simulink model "warning_system_harness"  (R2024b)
settings: Solver=FixedStepAuto  StartTime=0.0  StopTime=1500  FixedStep=TS_MODEL  RelTol=1e-3
InitFcn:
  | %run('config.m');
undefined symbols (not defined in the file or in its folder): THRESHOLD_CAUTION, THRESHOLD_CRASHED, THRESHOLD_LANE_CHANGE, THRESHOLD_REST, TS_CORE
libraries: dspstat3 x3, simulink x3, SignalEditorBlockLib x1
settings Model: DataDictionary=try__.sldd  SimulationMode=rapid-accelerator  ExtModeTrigDuration=2  Creator=Nitesh  LastModifiedBy=Nitesh
settings SolverCC: AutoInsertRateTranBlk=on
settings OptimizationCC: EnhancedBackFolding=on  PassReuseOutputArgsAs=Individual arguments  ZeroExternalMemoryAtStartup=off  ZeroInternalMemoryAtStartup=off  MaxStackSize=64  OptimizeBlockOrder=speed  DifferentSizesBufferReuse=on  OptimizationCustomize=off  EfficientTunableParamExpr=on
settings DebuggingCC: ParameterTunabilityLossMsg=error
settings HardwareCC: ProdBitPerPointer=32  ProdBitPerSizeT=32  ProdBitPerPtrDiffT=32  ProdLargestAtomicInteger=Long  ProdLargestAtomicFloat=Double  ProdWordSize=32  ProdHWDeviceType=ARM Compatible->ARM Cortex  UseEmbeddedCoderFeatures=off
settings RTWCC: Description=Embedded Coder  SystemTargetFile=ert.tlc  HardwareBoard=ESP32-WROOM(Arduino Compatible)  TLCOptions="-aInlineSetEventsForThisBaseRateFcn=TLC_FALSE -aSuppressMultiTaskScheduler=TLC_FALSE  -aRateBasedStepFcn=0"  TemplateMakefile=ert_default_tmf  Toolchain=ESP32
settings CodeAppCC: ForceParamTrailComments=on  IgnoreCustomStorageClasses=off  OperatorAnnotations=on  SimulinkDataObjDesc=on  SFDataObjDesc=on  InsertBlockDesc=on
settings ERTTargetCC: MultiwordLength=2048  DynamicStringBufferSize=2048  SupportContinuousTime=on  SupportNonInlinedSFcns=on  SupportVariableSizeSignals=on  ExtModeTransport=3  ExtModeStaticAlloc=on  ExtModeAutomaticAllocSize=off  ExtModeStaticAllocSize=65536  ExtModeMexFile=ext_xcp  ExtModeIntrfLevel=Level2 - Open  InlinedParameterPlacement=Hierarchical

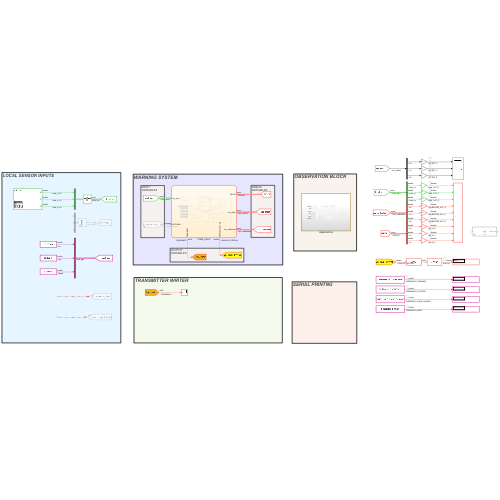
[thumbnail: Simulink's stored preview of the top-level diagram]
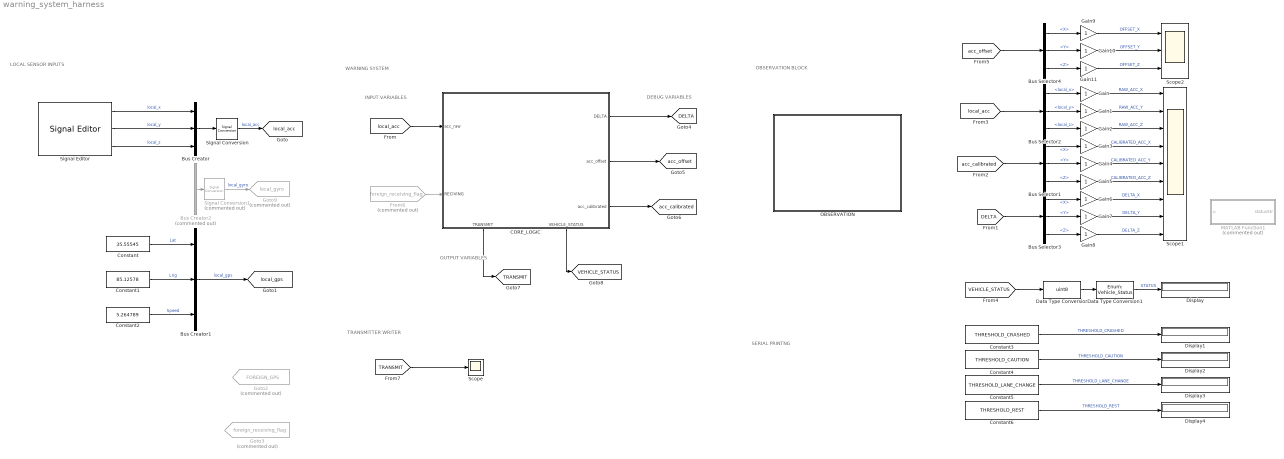
== system warning_system_harness ==
  note: SERIAL PRINTNG
  note: DEBUG
      | VARIABLES
  note: OBSERVATION BLOCK
  note: TRANSMITTER WRITER
  note: WARNING SYSTEM
  note: LOCAL SENSOR INPUTS
  note: OUTPUT
      | VARIABLES
  note: INPUT
      | VARIABLES
  Bus Creator : BusCreator  Inputs=3
  Bus Creator1 : BusCreator  Inputs=3
  Bus Creator2 : BusCreator  Commented=on  Inputs=3
  Bus Selector1 : BusSelector  OutputSignals=X,Y,Z
  Bus Selector2 : BusSelector  OutputSignals=local_x,local_y,local_z
  Bus Selector3 : BusSelector  OutputSignals=X,Y,Z
  Bus Selector4 : BusSelector  OutputSignals=X,Y,Z
  CORE_LOGIC : Stateflow chart  TreatAsAtomicUnit=on  SystemSampleTime=TS_CORE
      settings: PortSchema="{\"entries\":[{\"content\":{\"sides\":[{\"content\":{\"connectorIds\":[\"In2\",\"In1\"]},\"type\":\"ConnectorPlacement.EquallySpacedRectSide\",\"uuid\":\"ee7c9145-97fe-42bf-b38f-25095debb339\"},{\"content\":{\"connectorIds\":[\"Out2\",\"Out3\",\"Out4\"],\"side\":\"RIGHT\"},\"type\":\"ConnectorPlacement.EquallySpacedRectSide\",\"uuid\":\"6ad3cc48-74a8-47e1-8b84-b3331846d199\"},{\"content\":{\"side\":\"TOP\"},\"type\":\"ConnectorPlacement.EquallySpacedRectSide\",\"uuid\":\"0e80e778-40c2-414e-b172-27c343627a22\"},{\"content\":{\"connectorIds\":[\"Out1\",\"Out5\"],\"side\":\"BOTTOM\"},\"type\":\"ConnectorPlacement.EquallySpacedRectSide\",\"uuid\":\"8c076511-fb77-4abd-9a6c-f32e2686fd08\"}]},\"type\":\"ConnectorPlacement.EquallySpacedConnector\",\"uuid\":\"44f6d062-1c8f-4774-b93e-5476bfb914ed\"}],\"packageUris\":[\"http://schema.mathworks.com/mf0/Connector/R2020b\"],\"version\":\"1.0\"}"
  Constant : Constant  Value=35.55545
  Constant1 : Constant  Value=85.12578
  Constant2 : Constant  Value=5.264789
  Constant3 : Constant  Value=THRESHOLD_CRASHED
  Constant4 : Constant  Value=THRESHOLD_CAUTION
  Constant5 : Constant  Value=THRESHOLD_LANE_CHANGE
  Constant6 : Constant  Value=THRESHOLD_REST
  Data Type Conversion : DataTypeConversion  OutDataTypeStr=uint8  SaturateOnIntegerOverflow=off  RndMeth=Floor
  Data Type Conversion1 : DataTypeConversion  OutDataTypeStr=Enum: Vehicle_Status  SaturateOnIntegerOverflow=off  RndMeth=Floor
  Display{,1..4} (5 alike) : Display
  From6 : From  Commented=on  GotoTag=foreign_receiving_flag  TagVisibility=global
  Gain{,1..11} (12 alike) : Gain
  Goto2 : Goto  Commented=on  GotoTag=FOREIGN_GPS  TagVisibility=global
  Goto3 : Goto  Commented=on  GotoTag=foreign_receiving_flag  TagVisibility=global
  Goto9 : Goto  Commented=on  GotoTag=local_gyro  TagVisibility=global
  MATLAB Function1 : MATLAB Function  Commented=on  TreatAsAtomicUnit=on
  OBSERVATION : Subsystem
  Scope : Scope
  Scope1 : Scope  NumInputPorts=9
  Scope2 : Scope  NumInputPorts=3
  Signal Conversion : SignalConversion  ConversionOutput=Nonvirtual bus  OutDataTypeStr=Bus: accel  OverrideOpt=off
  Signal Conversion1 : SignalConversion  Commented=on  ConversionOutput=Nonvirtual bus  OutDataTypeStr=Bus: accel  OverrideOpt=off
  Signal Editor : SignalEditorBlockLib/Signal Editor  FileName=acc_data.mat  ActiveScenario=ash_car  ActiveSignal=X  IsBus=off  OutputBusObjectStr=Bus: BusObject  SampleTime=0.1  Interpolate=off  ZeroCross=off  OutputAfterFinalValue=Setting to zero  Unit=inherit  PreserveSignalName=on  ApplySigPropsToAllScenarios=on  ApplySigPropsToAllSignals=on
  tag scope: DELTA=global, TRANSMIT=global, VEHICLE_STATUS=global, acc_calibrated=global, acc_offset=global, local_acc=global, local_gps=global
  wires:
  Signal Editor/1 -> Bus Creator/1  "local_x"
  Signal Editor/2 -> Bus Creator/2  "local_y"
  Signal Editor/3 -> Bus Creator/3  "local_z"
  Bus Creator/1 -> Signal Conversion/1
  [local_acc] -> CORE_LOGIC/2(acc_raw)
  Bus Creator1/1 -> [local_gps]  "local_gps"
  ? -> Goto2/1
  ? -> Goto3/1
  From6/1 -> CORE_LOGIC/1(RECIVING)
  CORE_LOGIC/2(DELTA) -> [DELTA]
  CORE_LOGIC/3(acc_offset) -> [acc_offset]
  CORE_LOGIC/4(acc_calibrated) -> [acc_calibrated]
  CORE_LOGIC/5(VEHICLE_STATUS) -> [VEHICLE_STATUS]
  CORE_LOGIC/1(TRANSMIT) -> [TRANSMIT]
  [TRANSMIT] -> Scope/1
  Bus Creator2/1 -> Signal Conversion1/1
  Constant/1 -> Bus Creator1/1  "Lat"
  Constant1/1 -> Bus Creator1/2  "Lng"
  Constant2/1 -> Bus Creator1/3  "Speed"
  Signal Conversion/1 -> [local_acc]  "local_acc"
  Signal Conversion1/1 -> Goto9/1  "local_gyro"
  [local_acc] -> Bus Selector2/1
  Bus Selector2/1 -> Gain/1  "<local_x>"
  Bus Selector2/3 -> Gain2/1  "<local_z>"
  Bus Selector2/2 -> Gain1/1  "<local_y>"
  Gain2/1 -> Scope1/3  "RAW_ACC_Z"
  Gain1/1 -> Scope1/2  "RAW_ACC_Y"
  Gain/1 -> Scope1/1  "RAW_ACC_X"
  Bus Selector1/2 -> Gain4/1  "<Y>"
  Bus Selector1/3 -> Gain5/1  "<Z>"
  Bus Selector1/1 -> Gain3/1  "<X>"
  [acc_calibrated] -> Bus Selector1/1
  [DELTA] -> Bus Selector3/1
  Bus Selector3/1 -> Gain6/1  "<X>"
  Bus Selector3/3 -> Gain8/1  "<Z>"
  Bus Selector3/2 -> Gain7/1  "<Y>"
  Gain3/1 -> Scope1/4  "CALIBRATED_ACC_X"
  Gain4/1 -> Scope1/5  "CALIBRATED_ACC_Y"
  Gain5/1 -> Scope1/6  "CALIBRATED_ACC_Z"
  Gain6/1 -> Scope1/7  "DELTA_X"
  Gain7/1 -> Scope1/8  "DELTA_Y"
  Gain8/1 -> Scope1/9  "DELTA_Z"
  [VEHICLE_STATUS] -> Data Type Conversion/1
  Data Type Conversion/1 -> Data Type Conversion1/1
  Data Type Conversion1/1 -> Display/1  "STATUS"
  Constant3/1 -> Display1/1  "THRESHOLD_CRASHED"
  Constant6/1 -> Display4/1  "THRESHOLD_REST"
  Constant5/1 -> Display3/1  "THRESHOLD_LANE_CHANGE"
  Constant4/1 -> Display2/1  "THRESHOLD_CAUTION"
  [acc_offset] -> Bus Selector4/1
  Bus Selector4/1 -> Gain9/1  "<X>"
  Bus Selector4/2 -> Gain10/1  "<Y>"
  Bus Selector4/3 -> Gain11/1  "<Z>"
  Gain9/1 -> Scope2/1  "OFFSET_X"
  Gain11/1 -> Scope2/3  "OFFSET_Z"
  Gain10/1 -> Scope2/2  "OFFSET_Y"

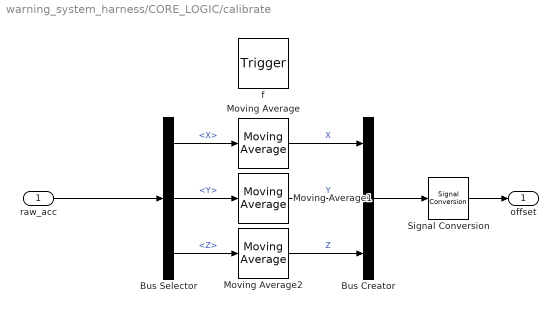
== system warning_system_harness/CORE_LOGIC/calibrate ==
  raw_acc : Inport  OutDataTypeStr=Bus: accel  PortDimensions=1
  f : TriggerPort  TriggerType=function-call  VariantControl=(inherit)
      settings: CopyFcn=Stateflow.SLINSF.SimulinkMan.removeBlockPreDeleteFcn  PreDeleteFcn=Stateflow.SLINSF.SimulinkMan.unsafePredeleteFcn
  Bus Creator : BusCreator  Inputs=3  OutDataTypeStr=Bus: accel
  Bus Selector : BusSelector  OutputSignals=X,Y,Z
  Moving Average : dspstat3/Moving Average  Method=Sliding window  ForgettingFactorPort=off  SpecifyWindowLength=on  WindowLength=4  OverlapLength=3  AllowArbitraryInputLength=off  ForgettingFactor=0.9  SimulateUsing=Code generation
  Moving Average1 : dspstat3/Moving Average  Method=Sliding window  ForgettingFactorPort=off  SpecifyWindowLength=on  WindowLength=4  OverlapLength=3  AllowArbitraryInputLength=off  ForgettingFactor=0.9  SimulateUsing=Code generation
  Moving Average2 : dspstat3/Moving Average  Method=Sliding window  ForgettingFactorPort=off  SpecifyWindowLength=on  WindowLength=4  OverlapLength=3  AllowArbitraryInputLength=off  ForgettingFactor=0.9  SimulateUsing=Code generation
  Signal Conversion : SignalConversion  ConversionOutput=Nonvirtual bus  OutDataTypeStr=Bus: accel  OverrideOpt=off
  offset : Outport  OutDataTypeStr=Bus: accel
  wires:
  raw_acc/1 -> Bus Selector/1
  Bus Selector/1 -> Moving Average/1  "<X>"
  Bus Selector/2 -> Moving Average1/1  "<Y>"
  Bus Selector/3 -> Moving Average2/1  "<Z>"
  Moving Average/1 -> Bus Creator/1  "X"
  Moving Average1/1 -> Bus Creator/2  "Y"
  Moving Average2/1 -> Bus Creator/3  "Z"
  Bus Creator/1 -> Signal Conversion/1
  Signal Conversion/1 -> offset/1

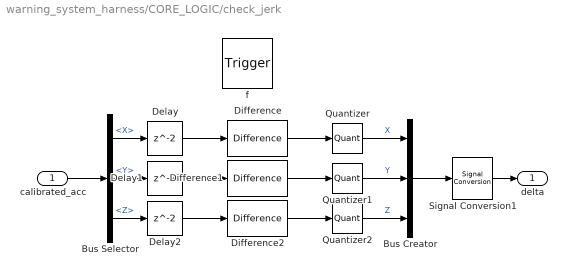
== system warning_system_harness/CORE_LOGIC/check_jerk ==
  calibrated_acc : Inport  OutDataTypeStr=Bus: accel  PortDimensions=1
  f : TriggerPort  TriggerType=function-call  VariantControl=(inherit)
      settings: CopyFcn=Stateflow.SLINSF.SimulinkMan.removeBlockPreDeleteFcn  PreDeleteFcn=Stateflow.SLINSF.SimulinkMan.unsafePredeleteFcn
  Bus Creator : BusCreator  Inputs=3  OutDataTypeStr=Bus: accel
  Bus Selector : BusSelector  OutputSignals=X,Y,Z
  Delay : Delay
  Delay1 : Delay
  Delay2 : Delay
  Difference : simulink/Discrete/Difference  ICPrevInput=0.0  OutMin=[]  OutMax=[]  OutDataType=fixdt(1, 16)  OutScaling=2^-10  DoSatur=off
  Difference1 : simulink/Discrete/Difference  ICPrevInput=0.0  OutMin=[]  OutMax=[]  OutDataType=fixdt(1, 16)  OutScaling=2^-10  DoSatur=off
  Difference2 : simulink/Discrete/Difference  ICPrevInput=0.0  OutMin=[]  OutMax=[]  OutDataType=fixdt(1, 16)  OutScaling=2^-10  DoSatur=off
  Quantizer : Quantizer  QuantizationInterval=0.1
  Quantizer1 : Quantizer  QuantizationInterval=0.1
  Quantizer2 : Quantizer  QuantizationInterval=0.1
  Signal Conversion1 : SignalConversion  ConversionOutput=Nonvirtual bus  OutDataTypeStr=Bus: accel  OverrideOpt=off
  delta : Outport  OutDataTypeStr=Bus: accel
  wires:
  Delay/1 -> Difference/1
  Difference/1 -> Quantizer/1
  calibrated_acc/1 -> Bus Selector/1
  Bus Selector/1 -> Delay/1  "<X>"
  Quantizer/1 -> Bus Creator/1  "X"
  Quantizer1/1 -> Bus Creator/2  "Y"
  Bus Selector/2 -> Delay1/1  "<Y>"
  Difference1/1 -> Quantizer1/1
  Delay1/1 -> Difference1/1
  Delay2/1 -> Difference2/1
  Difference2/1 -> Quantizer2/1
  Bus Selector/3 -> Delay2/1  "<Z>"
  Quantizer2/1 -> Bus Creator/3  "Z"
  Bus Creator/1 -> Signal Conversion1/1
  Signal Conversion1/1 -> delta/1

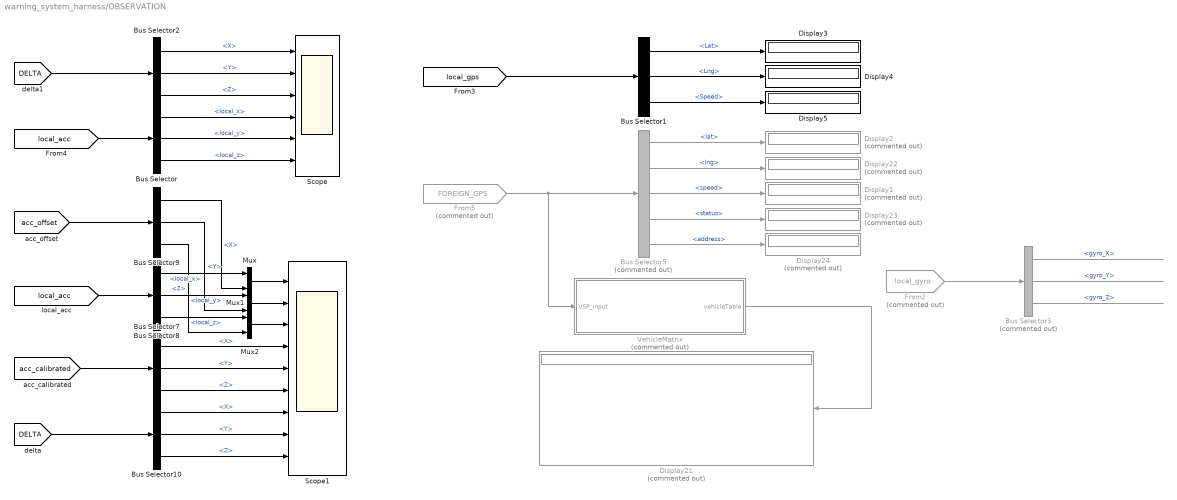
== system warning_system_harness/OBSERVATION ==
  Bus Selector : BusSelector  OutputSignals=local_x,local_y,local_z
  Bus Selector1 : BusSelector  OutputSignals=Lat,Lng,Speed
  Bus Selector{2,7,9..10} (4 alike) : BusSelector  OutputSignals=X,Y,Z
  Bus Selector3 : BusSelector  Commented=on  OutputSignals=gyro_X,gyro_Y,gyro_Z
  Bus Selector5 : BusSelector  Commented=on  OutputSignals=lat,lng,speed,status,address
  Bus Selector8 : BusSelector  OutputSignals=local_x,local_y,local_z
  Display{1..2,21..24} (6 alike) : Display  Commented=on
  Display3 : Display
  Display4 : Display
  Display5 : Display
  From2 : From  Commented=on  GotoTag=local_gyro  TagVisibility=global
  From5 : From  Commented=on  GotoTag=FOREIGN_GPS  TagVisibility=global
  Mux : Mux  Inputs=2
  Mux1 : Mux  Inputs=2
  Mux2 : Mux  Inputs=2
  Scope : Scope  NumInputPorts=6
  Scope1 : Scope  NumInputPorts=9
  VehicleMatrix : MATLAB Function  Commented=on  TreatAsAtomicUnit=on
  wires:
  [local_acc] -> Bus Selector/1
  Bus Selector/1 -> Scope/4  "<local_x>"
  Bus Selector/2 -> Scope/5  "<local_y>"
  Bus Selector/3 -> Scope/6  "<local_z>"
  Bus Selector5/1 -> Display2/1  "<lat>"
  Bus Selector5/2 -> Display22/1  "<lng>"
  Bus Selector5/3 -> Display1/1  "<speed>"
  Bus Selector5/4 -> Display23/1  "<status>"
  Bus Selector5/5 -> Display24/1  "<address>"
  VehicleMatrix/1(vehicleTable) -> Display21/1
  From5/1 -> VehicleMatrix/1(VSP_input), Bus Selector5/1
  [acc_calibrated] -> Bus Selector7/1
  [local_acc] -> Bus Selector8/1
  [acc_offset] -> Bus Selector9/1
  Mux/1 -> Scope1/1
  Mux2/1 -> Scope1/3
  Bus Selector8/1 -> Mux/1  "<local_x>"
  Bus Selector8/2 -> Mux1/1  "<local_y>"
  Bus Selector8/3 -> Mux2/1  "<local_z>"
  Bus Selector9/1 -> Mux/2  "<X>"
  Bus Selector9/2 -> Mux1/2  "<Y>"
  Bus Selector9/3 -> Mux2/2  "<Z>"
  Mux1/1 -> Scope1/2
  Bus Selector7/1 -> Scope1/4  "<X>"
  Bus Selector7/2 -> Scope1/5  "<Y>"
  Bus Selector7/3 -> Scope1/6  "<Z>"
  [DELTA] -> Bus Selector10/1
  Bus Selector10/1 -> Scope1/7  "<X>"
  Bus Selector10/2 -> Scope1/8  "<Y>"
  Bus Selector10/3 -> Scope1/9  "<Z>"
  [local_gps] -> Bus Selector1/1
  Bus Selector1/3 -> Display5/1  "<Speed>"
  Bus Selector1/1 -> Display3/1  "<Lat>"
  Bus Selector1/2 -> Display4/1  "<Lng>"
  [DELTA] -> Bus Selector2/1
  Bus Selector2/1 -> Scope/1  "<X>"
  Bus Selector2/2 -> Scope/2  "<Y>"
  Bus Selector2/3 -> Scope/3  "<Z>"
  From2/1 -> Bus Selector3/1
  Bus Selector3/3 -> ?  "<gyro_Z>"
  Bus Selector3/1 -> ?  "<gyro_X>"
  Bus Selector3/2 -> ?  "<gyro_Y>"

== matlab function warning_system_harness/MATLAB Function1 ==
  data: u input; statusStr output string
function statusStr = fcn(u)

    switch u
        case 0
            statusStr = "INVALID";
        case 4
            statusStr = 'NORMAL';
        case 8
            statusStr = 'LANE_CHANGE_RIGHT';
        case 16
            statusStr = 'LANE_CHANGE_LEFT';
        case 32
            statusStr = 'NEARBY_CRASH';
        case 128
            statusStr = 'CRASH';
        case 100
            statusStr = 'CAUTION';
        otherwise
            statusStr = 'UNKNOWN';
    end

== stateflow chart warning_system_harness/CORE_LOGIC ==
  state Init
    en:
    COUNT_CALIBRATION = 10;
    VEHICLE_STATUS=8;
    COUNT_CRASHED=0;
    COUNT_NEARBY_CRASHED=0;
    COUNT_CAUTION=0;
    TRANSMIT = 0;
  state MPU_Running
    state Extracting_Values
      during:
      acc_calibrated.X =  acc_raw.X - acc_offset.X;
      acc_calibrated.Y =  acc_raw.Y - acc_offset.Y;
      acc_calibrated.Z =  acc_raw.Z - acc_offset.Z;
    state jerk_check
      en:
      DELTA = check_jerk(acc_calibrated);
    (default) -> Extracting_Values
    Extracting_Values -> jerk_check [order 3] : [temporalCount(tick)>1]
  state caliberation
    en:
    acc_offset =   calibrate(acc_raw);
  state normal
    entry:
    VEHICLE_STATUS=4;
    if (TRANSMIT>0)
    TRANSMIT = TRANSMIT-1;
    end
    if (lane_changed==1)
    %RIGHT
    VEHICLE_STATUS =8;
    TRANSMIT = 8;
    elseif (lane_changed==-1)
    %LEFT
    VEHICLE_STATUS =16;
    TRANSMIT = 8;
    end
  state delta = check_jerk(calibrated_acc) [function]
  state caution
    en:
    VEHICLE_STATUS=100;
  state crashed
    entry:
    VEHICLE_STATUS=128;
  state nearby_crash
    entry:
    VEHICLE_STATUS=32;
  state offset = calibrate(raw_acc) [function]
  Extracting_Values -> (junction 43) [order 1] : [is_rest && OFFSET_MISMATCH(COUNT_CALIBRATION)]
  (junction 43) -> caliberation
  (default) -> Init
  Init -> MPU_Running
  Extracting_Values -> (junction 40) [order 2] : [COUNT_CALIBRATION>0]
      | {COUNT_CALIBRATION = COUNT_CALIBRATION - 1}
  (junction 40) -> caliberation
  caliberation -> (junction 35)
  (junction 35) -> MPU_Running
  (junction 103) -> MPU_Running
  (junction 102) -> (junction 103)
  jerk_check -> (junction 142) [order 3] : [COUNT_CRASHED>4]
  (junction 142) -> crashed
  jerk_check -> (junction 145) [order 2] : [is_crashed]
  (junction 145) -> crashed : {COUNT_CRASHED = 15;}
  jerk_check -> (junction 154) [order 4] : [COUNT_NEARBY_CRASHED>10]
  (junction 154) -> nearby_crash
  jerk_check -> (junction 167) [order 6] : [COUNT_CAUTION>5]
  (junction 167) -> caution
  jerk_check -> (junction 148) [order 1] : [RECIVING==true]
  jerk_check -> (junction 181) [order 5]
  (junction 148) -> nearby_crash : {COUNT_NEARBY_CRASHED = 8}
  (junction 181) -> caution : [is_caution]
      | {COUNT_CRASHED=7}
  jerk_check -> normal [order 7]
  caution -> (junction 161) : {
      | COUNT_CAUTION = COUNT_CAUTION-1;
      | TRANSMIT=COUNT_CAUTION;
      | }
  crashed -> (junction 97) : {
      | COUNT_CRASHED = COUNT_CRASHED-1;
      | TRANSMIT=COUNT_CRASHED;
      | }
  nearby_crash -> (junction 93) : {
      | COUNT_NEARBY_CRASHED = COUNT_NEARBY_CRASHED-1
      | TRANSMIT = COUNT_NEARBY_CRASHED
      | }
  normal -> (junction 96)
  (junction 93) -> (junction 102)
  (junction 96) -> (junction 93)
  (junction 161) -> (junction 96)
  (junction 97) -> (junction 161)
  data: COUNT_CALIBRATION function_input; count function_output; y function_output; y function_output; y function_output; y function_output; calibrated_acc function_input Bus: accel size=1; delta function_output Bus: accel; raw_acc function_input Bus: accel size=1; offset function_output Bus: accel; TRANSMIT output uint8; RECIVING input boolean; COUNT_CALIBRATION local uint8; THRESHOLD_REST parameter; THRESHOLD_CRASHED parameter; DELTA output Bus: accel size=1 =struct('X', 0, 'Y', 0, 'Z', 0); acc_offset output Bus: accel size=1 =struct('X', 0, 'Y', 0, 'Z', 0); acc_calibrated output Bus: accel size=1 =struct('X', 0, 'Y', 0, 'Z', 0); acc_raw input Bus: accel; VEHICLE_STATUS output; COUNT_CRASHED local uint8; COUNT_NEARBY_CRASHED local uint8; THRESHOLD_CAUTION parameter; THRESHOLD_LANE_CHANGE parameter; COUNT_CAUTION local uint8
  function count = OFFSET_MISMATCH(COUNT_CALIBRATION):
    | function count = OFFSET_MISMATCH(COUNT_CALIBRATION)
    | 
    | count = COUNT_CALIBRATION;
    | if(abs(acc_raw.X - acc_offset.X) > 0.01 && ...
    |    abs(acc_raw.Y - acc_offset.Y) > 0.01 && ...
    |    abs(acc_raw.Z - acc_offset.Z) > 0.01)
    | 
    |     count = COUNT_CALIBRATION +1;
    | end
  function y = lane_changed:
    | function y = lane_changed
    | 
    | y = 0;
    | 
    | if (acc_calibrated.X > THRESHOLD_LANE_CHANGE)
    |     % LEFT
    |     y = 1; 
    | elseif (acc_calibrated.X < -THRESHOLD_LANE_CHANGE)
    |     % RIGHT
    |     y = -1;
    | end
  function y = is_caution:
    | function y = is_caution
    |  
    | 
    | if (abs(DELTA.Y) >= THRESHOLD_CAUTION)
    |    
    |     y = true; 
    | else 
    |     y = false;
    | end
  function y = is_rest:
    | function y = is_rest
    | 
    | if (abs(DELTA.X) >= THRESHOLD_REST &&...
    |     abs(DELTA.Y) >= THRESHOLD_REST &&...
    |     abs(DELTA.Z) >= THRESHOLD_REST )
    |     y = true; 
    | else 
    |     y = false;
    | end
  function y = is_crashed:
    | function y = is_crashed
    | 
    | if (abs(DELTA.Y) >= THRESHOLD_CRASHED)
    |     y = true; 
    | else 
    |     y = false;
    | end

== matlab function warning_system_harness/OBSERVATION/VehicleMatrix ==
  data: VSP_input input; vehicleTable output size=[10, 5]
function vehicleTable = updateVehicleMatrix(VSP_input)
    %#codegen
    persistent table
    maxRows = 10;
    numCols = 5;

    if isempty(table)
        table = zeros(maxRows, numCols);  % Fixed size [10x5]
    end

    % Predeclare output for fixed-size requirement
    vehicleTable = zeros(maxRows, numCols);

    % Check if vehicle already exists — update if found
    for i = 1:maxRows
        if table(i, 1) == double(VSP_input.address)
            table(i, :) = [ ...
                double(VSP_input.address), ...
                double(VSP_input.status), ...
                VSP_input.lat, ...
                VSP_input.lng, ...
                VSP_input.speed];
            vehicleTable = table;
            return;
        end
    end

    % Try to insert into first empty row
    for i = 1:maxRows
        if table(i, 1) == 0
            table(i, :) = [ ...
                double(VSP_input.address), ...
                double(VSP_input.status), ...
                VSP_input.lat, ...
                VSP_input.lng, ...
                VSP_input.speed];
            vehicleTable = table;
            return;
        end
    end

    % If full, replace first row
    table(1, :) = [ ...
        double(VSP_input.address), ...
        double(VSP_input.status), ...
        VSP_input.lat, ...
        VSP_input.lng, ...
        VSP_input.speed];

    vehicleTable = table;
end
